simulink model "gm_DSBF"  (R2019b)
settings: Solver=FixedStepDiscrete  StartTime=0.0  StopTime=0.02  RelTol=1e-3
InitFcn:
  | sm_callback_init
StopFcn:
  | sm_callback_stop
undefined symbols (not defined in the file or in its folder): arraySize, arraySpacing, delayDataTypeFractionLength, delayDataTypeSign, delayDataTypeWordLength, mp, samplingRate, speedOfSound, upsampleFactor
libraries: hdlsllib x64, simulink x36, dspmlti4 x16, dsphdlfiltering x16
(part 5 of 5)

== system gm_DSBF/dataplane/Avalon Data Processing/delay signals_instance15/delay signal/read address generator/Subtract ==
  In1 : Inport  OutDataTypeStr=fixdt(1,6,0)
  In2 : Inport  Port=2  OutDataTypeStr=fixdt(0,6,0)
  In3 : Inport  Port=3  OutDataTypeStr=fixdt(0,6,0)
  Sum2 : Sum  AccumDataTypeStr=fixdt(1,8,0)  OutDataTypeStr=fixdt(1,8,0)
  Sum3 : Sum  Inputs=+-  AccumDataTypeStr=fixdt(1,8,0)  OutDataTypeStr=fixdt(0,6,0)
  Out1 : Outport
  wires:
  Sum3/1 -> Out1/1
  In3/1 -> Sum3/2
  Sum2/1 -> Sum3/1
  In2/1 -> Sum2/2
  In1/1 -> Sum2/1

== system gm_DSBF/dataplane/Avalon Data Processing/delay signals_instance15/delay signal/read address generator1/Subtract ==
  In1 : Inport  OutDataTypeStr=fixdt(1,6,0)
  In2 : Inport  Port=2  OutDataTypeStr=fixdt(0,6,0)
  In3 : Inport  Port=3  OutDataTypeStr=fixdt(0,6,0)
  Sum2 : Sum  AccumDataTypeStr=fixdt(1,8,0)  OutDataTypeStr=fixdt(1,8,0)
  Sum3 : Sum  Inputs=+-  AccumDataTypeStr=fixdt(1,8,0)  OutDataTypeStr=fixdt(0,6,0)
  Out1 : Outport
  wires:
  Sum3/1 -> Out1/1
  In3/1 -> Sum3/2
  Sum2/1 -> Sum3/1
  In2/1 -> Sum2/2
  In1/1 -> Sum2/1

== system gm_DSBF/dataplane/Avalon Data Processing/delay signals_instance16/delay signal/read address generator/Subtract ==
  In1 : Inport  OutDataTypeStr=fixdt(1,6,0)
  In2 : Inport  Port=2  OutDataTypeStr=fixdt(0,6,0)
  In3 : Inport  Port=3  OutDataTypeStr=fixdt(0,6,0)
  Sum2 : Sum  AccumDataTypeStr=fixdt(1,8,0)  OutDataTypeStr=fixdt(1,8,0)
  Sum3 : Sum  Inputs=+-  AccumDataTypeStr=fixdt(1,8,0)  OutDataTypeStr=fixdt(0,6,0)
  Out1 : Outport
  wires:
  Sum3/1 -> Out1/1
  In3/1 -> Sum3/2
  Sum2/1 -> Sum3/1
  In2/1 -> Sum2/2
  In1/1 -> Sum2/1

== system gm_DSBF/dataplane/Avalon Data Processing/delay signals_instance16/delay signal/read address generator1/Subtract ==
  In1 : Inport  OutDataTypeStr=fixdt(1,6,0)
  In2 : Inport  Port=2  OutDataTypeStr=fixdt(0,6,0)
  In3 : Inport  Port=3  OutDataTypeStr=fixdt(0,6,0)
  Sum2 : Sum  AccumDataTypeStr=fixdt(1,8,0)  OutDataTypeStr=fixdt(1,8,0)
  Sum3 : Sum  Inputs=+-  AccumDataTypeStr=fixdt(1,8,0)  OutDataTypeStr=fixdt(0,6,0)
  Out1 : Outport
  wires:
  Sum3/1 -> Out1/1
  In3/1 -> Sum3/2
  Sum2/1 -> Sum3/1
  In2/1 -> Sum2/2
  In1/1 -> Sum2/1

== system gm_DSBF/dataplane/Avalon Data Processing/delay signals_instance2/delay signal/read address generator/Subtract ==
  In1 : Inport  OutDataTypeStr=fixdt(1,6,0)
  In2 : Inport  Port=2  OutDataTypeStr=fixdt(0,6,0)
  In3 : Inport  Port=3  OutDataTypeStr=fixdt(0,6,0)
  Sum2 : Sum  AccumDataTypeStr=fixdt(1,8,0)  OutDataTypeStr=fixdt(1,8,0)
  Sum3 : Sum  Inputs=+-  AccumDataTypeStr=fixdt(1,8,0)  OutDataTypeStr=fixdt(0,6,0)
  Out1 : Outport
  wires:
  Sum3/1 -> Out1/1
  In3/1 -> Sum3/2
  Sum2/1 -> Sum3/1
  In2/1 -> Sum2/2
  In1/1 -> Sum2/1

== system gm_DSBF/dataplane/Avalon Data Processing/delay signals_instance2/delay signal/read address generator1/Subtract ==
  In1 : Inport  OutDataTypeStr=fixdt(1,6,0)
  In2 : Inport  Port=2  OutDataTypeStr=fixdt(0,6,0)
  In3 : Inport  Port=3  OutDataTypeStr=fixdt(0,6,0)
  Sum2 : Sum  AccumDataTypeStr=fixdt(1,8,0)  OutDataTypeStr=fixdt(1,8,0)
  Sum3 : Sum  Inputs=+-  AccumDataTypeStr=fixdt(1,8,0)  OutDataTypeStr=fixdt(0,6,0)
  Out1 : Outport
  wires:
  Sum3/1 -> Out1/1
  In3/1 -> Sum3/2
  Sum2/1 -> Sum3/1
  In2/1 -> Sum2/2
  In1/1 -> Sum2/1

== system gm_DSBF/dataplane/Avalon Data Processing/delay signals_instance3/delay signal/read address generator/Subtract ==
  In1 : Inport  OutDataTypeStr=fixdt(1,6,0)
  In2 : Inport  Port=2  OutDataTypeStr=fixdt(0,6,0)
  In3 : Inport  Port=3  OutDataTypeStr=fixdt(0,6,0)
  Sum2 : Sum  AccumDataTypeStr=fixdt(1,8,0)  OutDataTypeStr=fixdt(1,8,0)
  Sum3 : Sum  Inputs=+-  AccumDataTypeStr=fixdt(1,8,0)  OutDataTypeStr=fixdt(0,6,0)
  Out1 : Outport
  wires:
  Sum3/1 -> Out1/1
  In3/1 -> Sum3/2
  Sum2/1 -> Sum3/1
  In2/1 -> Sum2/2
  In1/1 -> Sum2/1

== system gm_DSBF/dataplane/Avalon Data Processing/delay signals_instance3/delay signal/read address generator1/Subtract ==
  In1 : Inport  OutDataTypeStr=fixdt(1,6,0)
  In2 : Inport  Port=2  OutDataTypeStr=fixdt(0,6,0)
  In3 : Inport  Port=3  OutDataTypeStr=fixdt(0,6,0)
  Sum2 : Sum  AccumDataTypeStr=fixdt(1,8,0)  OutDataTypeStr=fixdt(1,8,0)
  Sum3 : Sum  Inputs=+-  AccumDataTypeStr=fixdt(1,8,0)  OutDataTypeStr=fixdt(0,6,0)
  Out1 : Outport
  wires:
  Sum3/1 -> Out1/1
  In3/1 -> Sum3/2
  Sum2/1 -> Sum3/1
  In2/1 -> Sum2/2
  In1/1 -> Sum2/1

== system gm_DSBF/dataplane/Avalon Data Processing/delay signals_instance4/delay signal/read address generator/Subtract ==
  In1 : Inport  OutDataTypeStr=fixdt(1,6,0)
  In2 : Inport  Port=2  OutDataTypeStr=fixdt(0,6,0)
  In3 : Inport  Port=3  OutDataTypeStr=fixdt(0,6,0)
  Sum2 : Sum  AccumDataTypeStr=fixdt(1,8,0)  OutDataTypeStr=fixdt(1,8,0)
  Sum3 : Sum  Inputs=+-  AccumDataTypeStr=fixdt(1,8,0)  OutDataTypeStr=fixdt(0,6,0)
  Out1 : Outport
  wires:
  Sum3/1 -> Out1/1
  In3/1 -> Sum3/2
  Sum2/1 -> Sum3/1
  In2/1 -> Sum2/2
  In1/1 -> Sum2/1

== system gm_DSBF/dataplane/Avalon Data Processing/delay signals_instance4/delay signal/read address generator1/Subtract ==
  In1 : Inport  OutDataTypeStr=fixdt(1,6,0)
  In2 : Inport  Port=2  OutDataTypeStr=fixdt(0,6,0)
  In3 : Inport  Port=3  OutDataTypeStr=fixdt(0,6,0)
  Sum2 : Sum  AccumDataTypeStr=fixdt(1,8,0)  OutDataTypeStr=fixdt(1,8,0)
  Sum3 : Sum  Inputs=+-  AccumDataTypeStr=fixdt(1,8,0)  OutDataTypeStr=fixdt(0,6,0)
  Out1 : Outport
  wires:
  Sum3/1 -> Out1/1
  In3/1 -> Sum3/2
  Sum2/1 -> Sum3/1
  In2/1 -> Sum2/2
  In1/1 -> Sum2/1

== system gm_DSBF/dataplane/Avalon Data Processing/delay signals_instance5/delay signal/read address generator/Subtract ==
  In1 : Inport  OutDataTypeStr=fixdt(1,6,0)
  In2 : Inport  Port=2  OutDataTypeStr=fixdt(0,6,0)
  In3 : Inport  Port=3  OutDataTypeStr=fixdt(0,6,0)
  Sum2 : Sum  AccumDataTypeStr=fixdt(1,8,0)  OutDataTypeStr=fixdt(1,8,0)
  Sum3 : Sum  Inputs=+-  AccumDataTypeStr=fixdt(1,8,0)  OutDataTypeStr=fixdt(0,6,0)
  Out1 : Outport
  wires:
  Sum3/1 -> Out1/1
  In3/1 -> Sum3/2
  Sum2/1 -> Sum3/1
  In2/1 -> Sum2/2
  In1/1 -> Sum2/1

== system gm_DSBF/dataplane/Avalon Data Processing/delay signals_instance5/delay signal/read address generator1/Subtract ==
  In1 : Inport  OutDataTypeStr=fixdt(1,6,0)
  In2 : Inport  Port=2  OutDataTypeStr=fixdt(0,6,0)
  In3 : Inport  Port=3  OutDataTypeStr=fixdt(0,6,0)
  Sum2 : Sum  AccumDataTypeStr=fixdt(1,8,0)  OutDataTypeStr=fixdt(1,8,0)
  Sum3 : Sum  Inputs=+-  AccumDataTypeStr=fixdt(1,8,0)  OutDataTypeStr=fixdt(0,6,0)
  Out1 : Outport
  wires:
  Sum3/1 -> Out1/1
  In3/1 -> Sum3/2
  Sum2/1 -> Sum3/1
  In2/1 -> Sum2/2
  In1/1 -> Sum2/1

== system gm_DSBF/dataplane/Avalon Data Processing/delay signals_instance6/delay signal/read address generator/Subtract ==
  In1 : Inport  OutDataTypeStr=fixdt(1,6,0)
  In2 : Inport  Port=2  OutDataTypeStr=fixdt(0,6,0)
  In3 : Inport  Port=3  OutDataTypeStr=fixdt(0,6,0)
  Sum2 : Sum  AccumDataTypeStr=fixdt(1,8,0)  OutDataTypeStr=fixdt(1,8,0)
  Sum3 : Sum  Inputs=+-  AccumDataTypeStr=fixdt(1,8,0)  OutDataTypeStr=fixdt(0,6,0)
  Out1 : Outport
  wires:
  Sum3/1 -> Out1/1
  In3/1 -> Sum3/2
  Sum2/1 -> Sum3/1
  In2/1 -> Sum2/2
  In1/1 -> Sum2/1

== system gm_DSBF/dataplane/Avalon Data Processing/delay signals_instance6/delay signal/read address generator1/Subtract ==
  In1 : Inport  OutDataTypeStr=fixdt(1,6,0)
  In2 : Inport  Port=2  OutDataTypeStr=fixdt(0,6,0)
  In3 : Inport  Port=3  OutDataTypeStr=fixdt(0,6,0)
  Sum2 : Sum  AccumDataTypeStr=fixdt(1,8,0)  OutDataTypeStr=fixdt(1,8,0)
  Sum3 : Sum  Inputs=+-  AccumDataTypeStr=fixdt(1,8,0)  OutDataTypeStr=fixdt(0,6,0)
  Out1 : Outport
  wires:
  Sum3/1 -> Out1/1
  In3/1 -> Sum3/2
  Sum2/1 -> Sum3/1
  In2/1 -> Sum2/2
  In1/1 -> Sum2/1

== system gm_DSBF/dataplane/Avalon Data Processing/delay signals_instance7/delay signal/read address generator/Subtract ==
  In1 : Inport  OutDataTypeStr=fixdt(1,6,0)
  In2 : Inport  Port=2  OutDataTypeStr=fixdt(0,6,0)
  In3 : Inport  Port=3  OutDataTypeStr=fixdt(0,6,0)
  Sum2 : Sum  AccumDataTypeStr=fixdt(1,8,0)  OutDataTypeStr=fixdt(1,8,0)
  Sum3 : Sum  Inputs=+-  AccumDataTypeStr=fixdt(1,8,0)  OutDataTypeStr=fixdt(0,6,0)
  Out1 : Outport
  wires:
  Sum3/1 -> Out1/1
  In3/1 -> Sum3/2
  Sum2/1 -> Sum3/1
  In2/1 -> Sum2/2
  In1/1 -> Sum2/1

== system gm_DSBF/dataplane/Avalon Data Processing/delay signals_instance7/delay signal/read address generator1/Subtract ==
  In1 : Inport  OutDataTypeStr=fixdt(1,6,0)
  In2 : Inport  Port=2  OutDataTypeStr=fixdt(0,6,0)
  In3 : Inport  Port=3  OutDataTypeStr=fixdt(0,6,0)
  Sum2 : Sum  AccumDataTypeStr=fixdt(1,8,0)  OutDataTypeStr=fixdt(1,8,0)
  Sum3 : Sum  Inputs=+-  AccumDataTypeStr=fixdt(1,8,0)  OutDataTypeStr=fixdt(0,6,0)
  Out1 : Outport
  wires:
  Sum3/1 -> Out1/1
  In3/1 -> Sum3/2
  Sum2/1 -> Sum3/1
  In2/1 -> Sum2/2
  In1/1 -> Sum2/1

== system gm_DSBF/dataplane/Avalon Data Processing/delay signals_instance8/delay signal/read address generator/Subtract ==
  In1 : Inport  OutDataTypeStr=fixdt(1,6,0)
  In2 : Inport  Port=2  OutDataTypeStr=fixdt(0,6,0)
  In3 : Inport  Port=3  OutDataTypeStr=fixdt(0,6,0)
  Sum2 : Sum  AccumDataTypeStr=fixdt(1,8,0)  OutDataTypeStr=fixdt(1,8,0)
  Sum3 : Sum  Inputs=+-  AccumDataTypeStr=fixdt(1,8,0)  OutDataTypeStr=fixdt(0,6,0)
  Out1 : Outport
  wires:
  Sum3/1 -> Out1/1
  In3/1 -> Sum3/2
  Sum2/1 -> Sum3/1
  In2/1 -> Sum2/2
  In1/1 -> Sum2/1

== system gm_DSBF/dataplane/Avalon Data Processing/delay signals_instance8/delay signal/read address generator1/Subtract ==
  In1 : Inport  OutDataTypeStr=fixdt(1,6,0)
  In2 : Inport  Port=2  OutDataTypeStr=fixdt(0,6,0)
  In3 : Inport  Port=3  OutDataTypeStr=fixdt(0,6,0)
  Sum2 : Sum  AccumDataTypeStr=fixdt(1,8,0)  OutDataTypeStr=fixdt(1,8,0)
  Sum3 : Sum  Inputs=+-  AccumDataTypeStr=fixdt(1,8,0)  OutDataTypeStr=fixdt(0,6,0)
  Out1 : Outport
  wires:
  Sum3/1 -> Out1/1
  In3/1 -> Sum3/2
  Sum2/1 -> Sum3/1
  In2/1 -> Sum2/2
  In1/1 -> Sum2/1

== system gm_DSBF/dataplane/Avalon Data Processing/delay signals_instance9/delay signal/read address generator/Subtract ==
  In1 : Inport  OutDataTypeStr=fixdt(1,6,0)
  In2 : Inport  Port=2  OutDataTypeStr=fixdt(0,6,0)
  In3 : Inport  Port=3  OutDataTypeStr=fixdt(0,6,0)
  Sum2 : Sum  AccumDataTypeStr=fixdt(1,8,0)  OutDataTypeStr=fixdt(1,8,0)
  Sum3 : Sum  Inputs=+-  AccumDataTypeStr=fixdt(1,8,0)  OutDataTypeStr=fixdt(0,6,0)
  Out1 : Outport
  wires:
  Sum3/1 -> Out1/1
  In3/1 -> Sum3/2
  Sum2/1 -> Sum3/1
  In2/1 -> Sum2/2
  In1/1 -> Sum2/1

== system gm_DSBF/dataplane/Avalon Data Processing/delay signals_instance9/delay signal/read address generator1/Subtract ==
  In1 : Inport  OutDataTypeStr=fixdt(1,6,0)
  In2 : Inport  Port=2  OutDataTypeStr=fixdt(0,6,0)
  In3 : Inport  Port=3  OutDataTypeStr=fixdt(0,6,0)
  Sum2 : Sum  AccumDataTypeStr=fixdt(1,8,0)  OutDataTypeStr=fixdt(1,8,0)
  Sum3 : Sum  Inputs=+-  AccumDataTypeStr=fixdt(1,8,0)  OutDataTypeStr=fixdt(0,6,0)
  Out1 : Outport
  wires:
  Sum3/1 -> Out1/1
  In3/1 -> Sum3/2
  Sum2/1 -> Sum3/1
  In2/1 -> Sum2/2
  In1/1 -> Sum2/1

== matlab function gm_DSBF/dataplane/Avalon Data Processing/deserializer/deserializer ==
  data: valid_out output; data_in input; data_out output; valid_in input; channel_in input; arraySize parameter
function [valid_out, data_out] = deserialize(data_in, valid_in, channel_in, arraySize)
%#codegen
persistent data_out_temp
persistent data_out_reg

if isempty(data_out_temp)
    data_out_temp = fi(zeros(arraySize(1)*arraySize(2), 1), data_in.numerictype);
end
if isempty(data_out_reg)
    data_out_reg = fi(zeros(arraySize(1)*arraySize(2), 1), data_in.numerictype);
end

valid_out = false;
data_out = data_out_reg;


if valid_in
    data_out_temp(channel_in + 1) = data_in;
    if channel_in == length(data_out_temp) - 1
        valid_out = true;
        data_out_reg = data_out_temp;
    end
else
end

== matlab function gm_DSBF/dataplane/Avalon Data Processing/delay signals_instance2/delay signal/split_into_int_and_frac_parts/split_into_int_and_frac_parts ==
  data: delay input; integer_delay output; fractional_delay output; upsampleFactor parameter; delayDataTypeFractionLength parameter
function [integer_delay, fractional_delay] = split_delay_into_int_and_frac_parts(delay, upsampleFactor, delayDataTypeFractionLength)
%#codegen
% truncate the delay value to get the integer part
integer_delay = fix(delay);

% get the fractional part of the delay and
% convert it to an integer at the upsampled clock rate
fractional_delay_temp = delay - integer_delay;
fractional_delay_temp_upsampled = round(upsampleFactor * fractional_delay_temp);
fractional_delay = fi(fractional_delay_temp_upsampled, 1, delayDataTypeFractionLength, 0);
end

== matlab function gm_DSBF/dataplane/Avalon Data Processing/delay signals_instance1/delay signal/split_into_int_and_frac_parts/split_into_int_and_frac_parts ==
  data: delay input; integer_delay output; fractional_delay output; upsampleFactor parameter; delayDataTypeFractionLength parameter
function [integer_delay, fractional_delay] = split_delay_into_int_and_frac_parts(delay, upsampleFactor, delayDataTypeFractionLength)
%#codegen
% truncate the delay value to get the integer part
integer_delay = fix(delay);

% get the fractional part of the delay and
% convert it to an integer at the upsampled clock rate
fractional_delay_temp = delay - integer_delay;
fractional_delay_temp_upsampled = round(upsampleFactor * fractional_delay_temp);
fractional_delay = fi(fractional_delay_temp_upsampled, 1, delayDataTypeFractionLength, 0);
end

== matlab function gm_DSBF/dataplane/Avalon Data Processing/delay signals_instance3/delay signal/split_into_int_and_frac_parts/split_into_int_and_frac_parts ==
  data: delay input; integer_delay output; fractional_delay output; upsampleFactor parameter; delayDataTypeFractionLength parameter
function [integer_delay, fractional_delay] = split_delay_into_int_and_frac_parts(delay, upsampleFactor, delayDataTypeFractionLength)
%#codegen
% truncate the delay value to get the integer part
integer_delay = fix(delay);

% get the fractional part of the delay and
% convert it to an integer at the upsampled clock rate
fractional_delay_temp = delay - integer_delay;
fractional_delay_temp_upsampled = round(upsampleFactor * fractional_delay_temp);
fractional_delay = fi(fractional_delay_temp_upsampled, 1, delayDataTypeFractionLength, 0);
end

== matlab function gm_DSBF/dataplane/Avalon Data Processing/delay signals_instance4/delay signal/split_into_int_and_frac_parts/split_into_int_and_frac_parts ==
  data: delay input; integer_delay output; fractional_delay output; upsampleFactor parameter; delayDataTypeFractionLength parameter
function [integer_delay, fractional_delay] = split_delay_into_int_and_frac_parts(delay, upsampleFactor, delayDataTypeFractionLength)
%#codegen
% truncate the delay value to get the integer part
integer_delay = fix(delay);

% get the fractional part of the delay and
% convert it to an integer at the upsampled clock rate
fractional_delay_temp = delay - integer_delay;
fractional_delay_temp_upsampled = round(upsampleFactor * fractional_delay_temp);
fractional_delay = fi(fractional_delay_temp_upsampled, 1, delayDataTypeFractionLength, 0);
end

== matlab function gm_DSBF/dataplane/Avalon Data Processing/delay signals_instance5/delay signal/split_into_int_and_frac_parts/split_into_int_and_frac_parts ==
  data: delay input; integer_delay output; fractional_delay output; upsampleFactor parameter; delayDataTypeFractionLength parameter
function [integer_delay, fractional_delay] = split_delay_into_int_and_frac_parts(delay, upsampleFactor, delayDataTypeFractionLength)
%#codegen
% truncate the delay value to get the integer part
integer_delay = fix(delay);

% get the fractional part of the delay and
% convert it to an integer at the upsampled clock rate
fractional_delay_temp = delay - integer_delay;
fractional_delay_temp_upsampled = round(upsampleFactor * fractional_delay_temp);
fractional_delay = fi(fractional_delay_temp_upsampled, 1, delayDataTypeFractionLength, 0);
end

== matlab function gm_DSBF/dataplane/Avalon Data Processing/delay signals_instance6/delay signal/split_into_int_and_frac_parts/split_into_int_and_frac_parts ==
  data: delay input; integer_delay output; fractional_delay output; upsampleFactor parameter; delayDataTypeFractionLength parameter
function [integer_delay, fractional_delay] = split_delay_into_int_and_frac_parts(delay, upsampleFactor, delayDataTypeFractionLength)
%#codegen
% truncate the delay value to get the integer part
integer_delay = fix(delay);

% get the fractional part of the delay and
% convert it to an integer at the upsampled clock rate
fractional_delay_temp = delay - integer_delay;
fractional_delay_temp_upsampled = round(upsampleFactor * fractional_delay_temp);
fractional_delay = fi(fractional_delay_temp_upsampled, 1, delayDataTypeFractionLength, 0);
end

== matlab function gm_DSBF/dataplane/Avalon Data Processing/delay signals_instance7/delay signal/split_into_int_and_frac_parts/split_into_int_and_frac_parts ==
  data: delay input; integer_delay output; fractional_delay output; upsampleFactor parameter; delayDataTypeFractionLength parameter
function [integer_delay, fractional_delay] = split_delay_into_int_and_frac_parts(delay, upsampleFactor, delayDataTypeFractionLength)
%#codegen
% truncate the delay value to get the integer part
integer_delay = fix(delay);

% get the fractional part of the delay and
% convert it to an integer at the upsampled clock rate
fractional_delay_temp = delay - integer_delay;
fractional_delay_temp_upsampled = round(upsampleFactor * fractional_delay_temp);
fractional_delay = fi(fractional_delay_temp_upsampled, 1, delayDataTypeFractionLength, 0);
end

== matlab function gm_DSBF/dataplane/Avalon Data Processing/delay signals_instance8/delay signal/split_into_int_and_frac_parts/split_into_int_and_frac_parts ==
  data: delay input; integer_delay output; fractional_delay output; upsampleFactor parameter; delayDataTypeFractionLength parameter
function [integer_delay, fractional_delay] = split_delay_into_int_and_frac_parts(delay, upsampleFactor, delayDataTypeFractionLength)
%#codegen
% truncate the delay value to get the integer part
integer_delay = fix(delay);

% get the fractional part of the delay and
% convert it to an integer at the upsampled clock rate
fractional_delay_temp = delay - integer_delay;
fractional_delay_temp_upsampled = round(upsampleFactor * fractional_delay_temp);
fractional_delay = fi(fractional_delay_temp_upsampled, 1, delayDataTypeFractionLength, 0);
end

== matlab function gm_DSBF/dataplane/Avalon Data Processing/delay signals_instance9/delay signal/split_into_int_and_frac_parts/split_into_int_and_frac_parts ==
  data: delay input; integer_delay output; fractional_delay output; upsampleFactor parameter; delayDataTypeFractionLength parameter
function [integer_delay, fractional_delay] = split_delay_into_int_and_frac_parts(delay, upsampleFactor, delayDataTypeFractionLength)
%#codegen
% truncate the delay value to get the integer part
integer_delay = fix(delay);

% get the fractional part of the delay and
% convert it to an integer at the upsampled clock rate
fractional_delay_temp = delay - integer_delay;
fractional_delay_temp_upsampled = round(upsampleFactor * fractional_delay_temp);
fractional_delay = fi(fractional_delay_temp_upsampled, 1, delayDataTypeFractionLength, 0);
end

== matlab function gm_DSBF/dataplane/Avalon Data Processing/delay signals_instance10/delay signal/split_into_int_and_frac_parts/split_into_int_and_frac_parts ==
  data: delay input; integer_delay output; fractional_delay output; upsampleFactor parameter; delayDataTypeFractionLength parameter
function [integer_delay, fractional_delay] = split_delay_into_int_and_frac_parts(delay, upsampleFactor, delayDataTypeFractionLength)
%#codegen
% truncate the delay value to get the integer part
integer_delay = fix(delay);

% get the fractional part of the delay and
% convert it to an integer at the upsampled clock rate
fractional_delay_temp = delay - integer_delay;
fractional_delay_temp_upsampled = round(upsampleFactor * fractional_delay_temp);
fractional_delay = fi(fractional_delay_temp_upsampled, 1, delayDataTypeFractionLength, 0);
end

== matlab function gm_DSBF/dataplane/Avalon Data Processing/delay signals_instance11/delay signal/split_into_int_and_frac_parts/split_into_int_and_frac_parts ==
  data: delay input; integer_delay output; fractional_delay output; upsampleFactor parameter; delayDataTypeFractionLength parameter
function [integer_delay, fractional_delay] = split_delay_into_int_and_frac_parts(delay, upsampleFactor, delayDataTypeFractionLength)
%#codegen
% truncate the delay value to get the integer part
integer_delay = fix(delay);

% get the fractional part of the delay and
% convert it to an integer at the upsampled clock rate
fractional_delay_temp = delay - integer_delay;
fractional_delay_temp_upsampled = round(upsampleFactor * fractional_delay_temp);
fractional_delay = fi(fractional_delay_temp_upsampled, 1, delayDataTypeFractionLength, 0);
end

== matlab function gm_DSBF/dataplane/Avalon Data Processing/delay signals_instance12/delay signal/split_into_int_and_frac_parts/split_into_int_and_frac_parts ==
  data: delay input; integer_delay output; fractional_delay output; upsampleFactor parameter; delayDataTypeFractionLength parameter
function [integer_delay, fractional_delay] = split_delay_into_int_and_frac_parts(delay, upsampleFactor, delayDataTypeFractionLength)
%#codegen
% truncate the delay value to get the integer part
integer_delay = fix(delay);

% get the fractional part of the delay and
% convert it to an integer at the upsampled clock rate
fractional_delay_temp = delay - integer_delay;
fractional_delay_temp_upsampled = round(upsampleFactor * fractional_delay_temp);
fractional_delay = fi(fractional_delay_temp_upsampled, 1, delayDataTypeFractionLength, 0);
end

== matlab function gm_DSBF/dataplane/Avalon Data Processing/delay signals_instance13/delay signal/split_into_int_and_frac_parts/split_into_int_and_frac_parts ==
  data: delay input; integer_delay output; fractional_delay output; upsampleFactor parameter; delayDataTypeFractionLength parameter
function [integer_delay, fractional_delay] = split_delay_into_int_and_frac_parts(delay, upsampleFactor, delayDataTypeFractionLength)
%#codegen
% truncate the delay value to get the integer part
integer_delay = fix(delay);

% get the fractional part of the delay and
% convert it to an integer at the upsampled clock rate
fractional_delay_temp = delay - integer_delay;
fractional_delay_temp_upsampled = round(upsampleFactor * fractional_delay_temp);
fractional_delay = fi(fractional_delay_temp_upsampled, 1, delayDataTypeFractionLength, 0);
end

== matlab function gm_DSBF/dataplane/Avalon Data Processing/delay signals_instance14/delay signal/split_into_int_and_frac_parts/split_into_int_and_frac_parts ==
  data: delay input; integer_delay output; fractional_delay output; upsampleFactor parameter; delayDataTypeFractionLength parameter
function [integer_delay, fractional_delay] = split_delay_into_int_and_frac_parts(delay, upsampleFactor, delayDataTypeFractionLength)
%#codegen
% truncate the delay value to get the integer part
integer_delay = fix(delay);

% get the fractional part of the delay and
% convert it to an integer at the upsampled clock rate
fractional_delay_temp = delay - integer_delay;
fractional_delay_temp_upsampled = round(upsampleFactor * fractional_delay_temp);
fractional_delay = fi(fractional_delay_temp_upsampled, 1, delayDataTypeFractionLength, 0);
end

== matlab function gm_DSBF/dataplane/Avalon Data Processing/delay signals_instance15/delay signal/split_into_int_and_frac_parts/split_into_int_and_frac_parts ==
  data: delay input; integer_delay output; fractional_delay output; upsampleFactor parameter; delayDataTypeFractionLength parameter
function [integer_delay, fractional_delay] = split_delay_into_int_and_frac_parts(delay, upsampleFactor, delayDataTypeFractionLength)
%#codegen
% truncate the delay value to get the integer part
integer_delay = fix(delay);

% get the fractional part of the delay and
% convert it to an integer at the upsampled clock rate
fractional_delay_temp = delay - integer_delay;
fractional_delay_temp_upsampled = round(upsampleFactor * fractional_delay_temp);
fractional_delay = fi(fractional_delay_temp_upsampled, 1, delayDataTypeFractionLength, 0);
end

== matlab function gm_DSBF/dataplane/Avalon Data Processing/delay signals_instance16/delay signal/split_into_int_and_frac_parts/split_into_int_and_frac_parts ==
  data: delay input; integer_delay output; fractional_delay output; upsampleFactor parameter; delayDataTypeFractionLength parameter
function [integer_delay, fractional_delay] = split_delay_into_int_and_frac_parts(delay, upsampleFactor, delayDataTypeFractionLength)
%#codegen
% truncate the delay value to get the integer part
integer_delay = fix(delay);

% get the fractional part of the delay and
% convert it to an integer at the upsampled clock rate
fractional_delay_temp = delay - integer_delay;
fractional_delay_temp_upsampled = round(upsampleFactor * fractional_delay_temp);
fractional_delay = fi(fractional_delay_temp_upsampled, 1, delayDataTypeFractionLength, 0);
end

== matlab function gm_DSBF/dataplane/Avalon Data Processing/normalize/normalize_shift/normalize_shift ==
  data: input input; normalized output
function normalized = fcn(input)
%#codegen
% NOTE: we should be normalizing to +/- 1 with the following commented line,
% but the AD1939 VHDL expects +/- 0.5 normalization; so for now, I'm 
% normalizing to +/- 0.5 until we fix the VHDL
%excessIntegerBits = input.WordLength - input.FractionLength - 1;
excessIntegerBits = input.WordLength - input.FractionLength;
normalized = bitsra(input, excessIntegerBits);
end

== matlab function gm_DSBF/dataplane/compute_delays/compute_delays ==
  data: sin_azimuth input; delays output; cos_elevation input; sin_elevation input; delayDataTypeSign parameter; delayDataTypeWordLength parameter; delayDataTypeFractionLength parameter; arraySize parameter; arraySpacing parameter; speedOfSound parameter; samplingRate parameter
function delays = computeDelays(sin_azimuth, cos_elevation, sin_elevation, delayDataTypeSign, delayDataTypeWordLength, delayDataTypeFractionLength, ...
    arraySize, arraySpacing, speedOfSound, samplingRate)
%#codegen    
ELEMENT_SPACING = fi(arraySpacing, 0, 16, 15);  % meters
SPEED_OF_SOUND = fi(speedOfSound, 0, 9, 0); % meters/second
NUM_ELEMENTS_Y = fi(arraySize(1), 1, 5, 1);
NUM_ELEMENTS_Z = fi(arraySize(2), 1, 5, 1);
SAMPLING_RATE = sfi(samplingRate);

delays = fi(zeros(arraySize(1) * arraySize(2), 1), delayDataTypeSign, delayDataTypeWordLength, delayDataTypeFractionLength);
yElementIdx = fi(0:(NUM_ELEMENTS_Y - 1), 1, 5, 1);
zElementIdx = fi((0:(NUM_ELEMENTS_Z - 1)), 1, 5, 1);

yDistanceFromPhaseCenter = ELEMENT_SPACING * (yElementIdx - (NUM_ELEMENTS_Y - 1)/2);
zDistanceFromPhaseCenter = ELEMENT_SPACING * (zElementIdx - (NUM_ELEMENTS_Z - 1)/2);

idx = fi(0, 0, log2(arraySize(1) * arraySize(2)) + 1, 0, 'SumMode', 'SpecifyPrecision', ...
    'SumWordLength', log2(arraySize(1) * arraySize(2)) + 1, 'SumFractionLength', 0);
for z = zElementIdx
    for y = yElementIdx
        idx = idx + 1;
        delays(idx) = -SAMPLING_RATE/SPEED_OF_SOUND  * (yDistanceFromPhaseCenter(y + 1) * sin_azimuth * cos_elevation + ...
            zDistanceFromPhaseCenter(z + 1) * sin_elevation);
    end
end
end
